simulink model "example_Test"  (R2015b)
settings: Solver=FixedStepAuto  StartTime=0.0  StopTime=10.0  FixedStep=0.1  RelTol=1e-3
libraries: realtime_pacer_lib x2
settings Model: Creator=shangwei  LastModifiedBy=shangwei

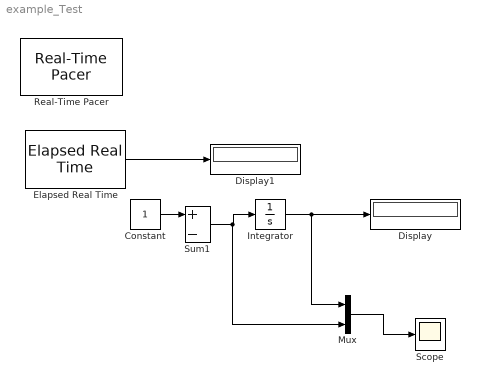
== system example_Test ==
  Constant : Constant
  Display : Display
  Display1 : Display
  Elapsed Real Time : realtime_pacer_lib/Elapsed Real Time
  Integrator : Integrator
  Mux : Mux  Inputs=2
  Real-Time Pacer : realtime_pacer_lib/Real-Time Pacer  simTimePerRealTime=1
  Scope : Scope
  Sum1 : Sum  Inputs=+-
  wires:
  Constant/1 -> Sum1/1
  Integrator/1 -> Mux/1, Display/1
  Elapsed Real Time/1 -> Display1/1
  Sum1/1 -> Mux/2, Integrator/1
  Mux/1 -> Scope/1
